simulink subsystem "CoulombCounting_Subsys"  (R2022b)
settings: Solver=VariableStepAuto  StartTime=0.0  StopTime=10.0  RelTol=1e-3
undefined symbols (not defined in the file): AH_TO_COULOMB, DiscIntNeverNeededParam, KeSoc_Ah_capacity, KeSoc_frc_SocMaxLim, KeSoc_frc_SocMinLim, SOC_CELLS_IN_PARALLEL
settings Model: Creator=Niharika  LastModifiedBy=Niharika

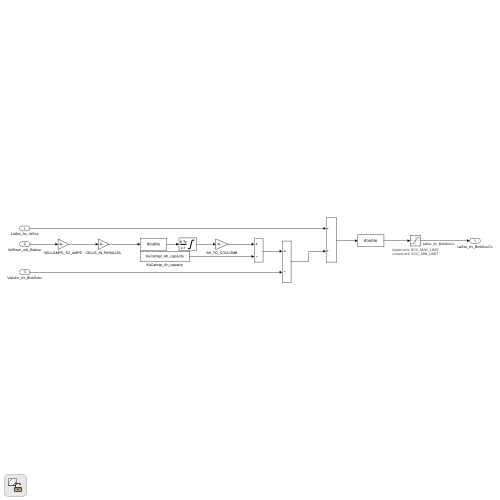
[thumbnail: Simulink's stored preview of the top-level diagram]
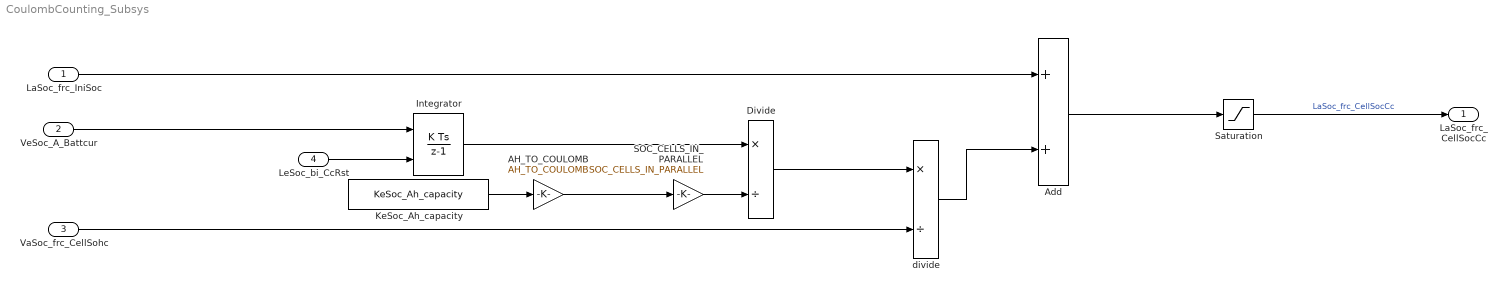
== system CoulombCounting_Subsys ==
  LaSoc_frc_IniSoc : Inport
  VeSoc_A_Battcur : Inport  Port=2
  VaSoc_frc_CellSohc : Inport  Port=3
  LeSoc_bi_CcRst : Inport  Port=4
  AH_TO_COULOMB : Gain  Gain=AH_TO_COULOMB
  Add : Sum
  Divide : Product  Inputs=*/
  Integrator : DiscreteIntegrator  gainval=1  ExternalReset=rising  SampleTime=-1  ICPrevOutput=DiscIntNeverNeededParam  ICPrevScaledInput=DiscIntNeverNeededParam
  KeSoc_Ah_capacity : Constant  Value=KeSoc_Ah_capacity  OutMin=0  OutMax=100
  SOC_CELLS_IN_PARALLEL : Gain  Gain=SOC_CELLS_IN_PARALLEL
  Saturation : Saturate  UpperLimit=KeSoc_frc_SocMaxLim  LowerLimit=KeSoc_frc_SocMinLim
      settings: AttributesFormatString=|
      | UpperLimit: %<UpperLimit>
      | LowerLimit: %<LowerLimit>
  divide : Product  Inputs=*/
  LaSoc_frc_CellSocCc : Outport
  wires:
  divide/1 -> Add/2
  Divide/1 -> divide/1
  LaSoc_frc_IniSoc/1 -> Add/1
  Saturation/1 -> LaSoc_frc_CellSocCc/1  "LaSoc_frc_CellSocCc"
  VaSoc_frc_CellSohc/1 -> divide/2
  Add/1 -> Saturation/1
  VeSoc_A_Battcur/1 -> Integrator/1
  KeSoc_Ah_capacity/1 -> AH_TO_COULOMB/1
  Integrator/1 -> Divide/1
  AH_TO_COULOMB/1 -> SOC_CELLS_IN_PARALLEL/1
  SOC_CELLS_IN_PARALLEL/1 -> Divide/2
  LeSoc_bi_CcRst/1 -> Integrator/2
